simulink model "smart_home"  (R2018b)
settings: Solver=VariableStepAuto  StartTime=0.0  StopTime=intervals  RelTol=1e-3
values from neighbouring files (symbols this model uses):
  bad_q = 300    [init.m]
  good_q = 100    [init.m]
  intervals = days*stepsInDay    (= 1152)    [init.m]
  stepsInDay = 24*60/timeStep    (= 288)    [init.m]
  sunrise = floor(0.25*stepsInDay)    [init.m]
  sunset = floor(0.8*stepsInDay)    [init.m]
  T_high = 24    [init.m]
  T_low = -5    [init.m]
libraries: simulink x8
settings Model: EnablePacing=on  PacingRate=10  Creator=jf  LastModifiedBy=jf
settings SolverCC: ZeroCrossControl=DisableAll

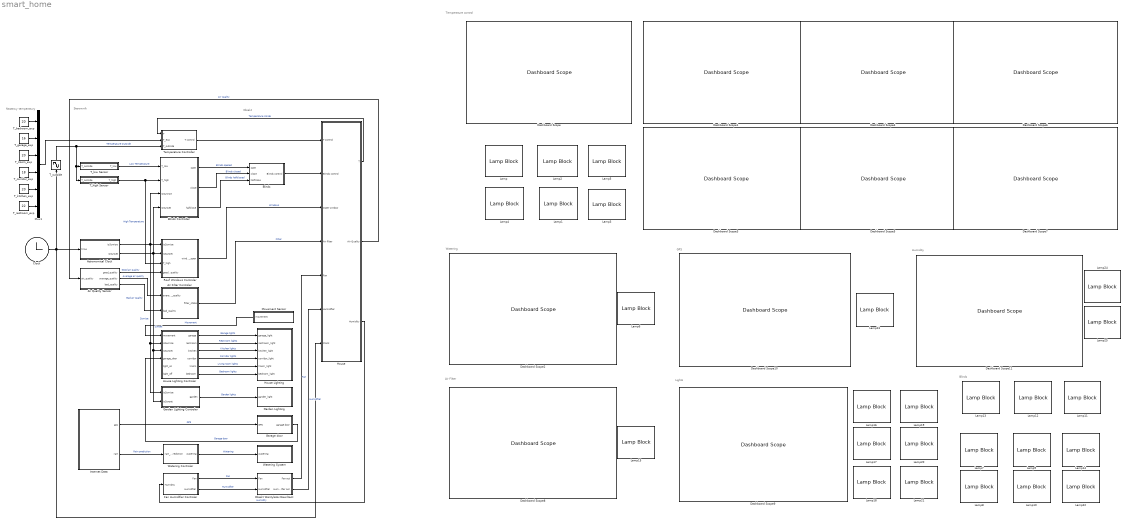
== system smart_home ==
  note: GPS
  note: Lights
  note: Air Filter
  note: Blinds
  note: Watering
  note: Temperature control
  note: Nastawy temperatury
  note: Sterownik
  note: Obiekt
  note: Humidity
  Air Filter Controler : Stateflow chart  TreatAsAtomicUnit=on
  Air Quality Sensor : Subsystem
  Astronomical Clock : Subsystem
  Blinds : Subsystem
  Blinds Controller : Stateflow chart  TreatAsAtomicUnit=on
  "Clock " : Clock
  Dashboard Scope : DashboardScope  WebBlockId=338  Ymax=30
  Dashboard Scope1 : DashboardScope  WebBlockId=352  Ymax=30
  Dashboard Scope10 : DashboardScope  WebBlockId=379  Ymin=-1  Ymax=1.5
  Dashboard Scope11 : DashboardScope  WebBlockId=384  Ymin=-1  Ymax=100
  Dashboard Scope2 : DashboardScope  WebBlockId=349  Ymin=-1  Ymax=1.5
  Dashboard Scope3 : DashboardScope  WebBlockId=353  Ymax=30
  Dashboard Scope4 : DashboardScope  WebBlockId=354  Ymax=30
  Dashboard Scope5 : DashboardScope  WebBlockId=355  Ymax=30
  Dashboard Scope6 : DashboardScope  WebBlockId=356  Ymax=30
  Dashboard Scope7 : DashboardScope  WebBlockId=357  Ymax=30
  Dashboard Scope8 : DashboardScope  WebBlockId=368  Ymin=-1  Ymax=1000
  Dashboard Scope9 : DashboardScope  WebBlockId=370  Ymin=-1  Ymax=8
  Fan Humidifier Controler : Subsystem
  Garage door : Subsystem
  Garden Lighting : Subsystem
  Garden Lighting Controler : Subsystem
  House : Subsystem
  House Lighting : Subsystem
  House Lighting Controler : Subsystem
  Internet Data : Subsystem
  Lamp : LampBlock  WebBlockId=341
  Lamp1 : LampBlock  WebBlockId=342
  Lamp10 : LampBlock  WebBlockId=361
  Lamp11 : LampBlock  WebBlockId=362
  Lamp12 : LampBlock  WebBlockId=363
  Lamp13 : LampBlock  WebBlockId=364
  Lamp14 : LampBlock  WebBlockId=366
  Lamp15 : LampBlock  WebBlockId=367
  Lamp16 : LampBlock  WebBlockId=371
  Lamp17 : LampBlock  WebBlockId=372
  Lamp18 : LampBlock  WebBlockId=373
  Lamp19 : LampBlock  WebBlockId=374
  Lamp2 : LampBlock  WebBlockId=343
  Lamp20 : LampBlock  WebBlockId=375
  Lamp21 : LampBlock  WebBlockId=376
  Lamp22 : LampBlock  WebBlockId=378
  Lamp23 : LampBlock  WebBlockId=380
  Lamp24 : LampBlock  WebBlockId=385
  Lamp25 : LampBlock  WebBlockId=387
  Lamp3 : LampBlock  WebBlockId=344
  Lamp4 : LampBlock  WebBlockId=345
  Lamp5 : LampBlock  WebBlockId=346
  Lamp6 : LampBlock  WebBlockId=350
  Lamp7 : LampBlock  WebBlockId=358
  Lamp8 : LampBlock  WebBlockId=359
  Lamp9 : LampBlock  WebBlockId=360
  Movement Sensor : Subsystem
  Mux1 : Mux  Inputs=6
  Obiekt Wentylator-Nawilzacz : Subsystem
  Roof Windows Controler : Subsystem
  T_bedroom_exp : Constant  Value=20
  T_corridor_exp : Constant  Value=18
  T_garage_exp : Constant  Value=16
  T_high Sensor : Subsystem
  T_kitchen_exp : Constant  Value=20
  T_low Sensor : Subsystem
  T_lroom_exp : Constant  Value=20
  T_outside : Sin  TimeSource=Use external signal  Amplitude=17  Bias=10  Frequency=2*pi/stepsInDay  Phase=-pi/2  SampleTime=0
  T_restroom_exp : Constant  Value=22
  Temperature Controller : Subsystem
  Watering Controler : Subsystem
  Watering System : Subsystem
  wires:
  T_high Sensor/1(T_high) -> Roof Windows Controler/3(T_high), Blinds Controller/2(T_high)  "High Temperature"
  T_garage_exp/1 -> Mux1/2
  "Clock "/1 -> Astronomical Clock/1(time), House/7(Clock), T_outside/1
  House Lighting Controler/4(corridor) -> House Lighting/4(corridor_light)  "Corridor lights"
  House Lighting Controler/5(lroom) -> House Lighting/5(lroom_light)  "Living room lights"
  Garden Lighting Controler/1(garden) -> Garden Lighting/1(garden_light)  "Garden lights"
  House Lighting Controler/1(garage) -> House Lighting/1(garage_light)  "Garage lights"
  House Lighting Controler/3(kitchen) -> House Lighting/3(kitchen_light)  "Kitchen lights"
  T_corridor_exp/1 -> Mux1/4
  T_restroom_exp/1 -> Mux1/6
  T_lroom_exp/1 -> Mux1/3
  T_bedroom_exp/1 -> Mux1/1
  T_kitchen_exp/1 -> Mux1/5
  House Lighting Controler/6(bedroom) -> House Lighting/6(bedroom_light)  "Bedroom lights"
  House Lighting Controler/2(restroom) -> House Lighting/2(restroom_light)  "Restroom lights"
  T_low Sensor/1(T_low) -> Blinds Controller/1(T_low)  "Low Temperature"
  Air Quality Sensor/1(good_quality) -> Roof Windows Controler/4(good_air_quality)  "Good air quality"
  Watering Controler/1(watering) -> Watering System/1(watering)  "Watering"
  Air Quality Sensor/2(avarage_quality) -> Air Filter Controler/1(average_quality)  "Avarage air quality"
  Air Quality Sensor/3(bad_quality) -> Air Filter Controler/2(bad_quality)  "Bad air quality"
  Blinds Controller/1(open) -> Blinds/1(open)  "Blinds opened"
  Blinds Controller/2(close) -> Blinds/2(close)  "Blinds closed"
  Blinds Controller/3(halfclose) -> Blinds/3(halfclose)  "Blinds halfclosed"
  Blinds/1(Blinds control) -> House/2(Blinds control)
  Roof Windows Controler/1(window_open) -> House/3(Open window)  "Windows"
  Air Filter Controler/1(filter_state) -> House/4(Air filter)  "Filter"
  House/1(T) -> Temperature Controller/1(T)  "Temperature inside"
  Temperature Controller/1(T control) -> House/1(T control)
  Mux1/1 -> Temperature Controller/2(T_exp)
  T_outside/1 -> T_high Sensor/1(T_outside), T_low Sensor/1(T_outside), Temperature Controller/3(T_outside)  "Temperature Outside"
  Internet Data/2(rain) -> Watering Controler/1(rain_prediction)  "Rain prediction"
  Internet Data/1(gps) -> Garage door/1(GPS)  "GPS"
  Astronomical Clock/1(isSunrise) -> Roof Windows Controler/1(isSunrise), Garden Lighting Controler/1(isSunrise), House Lighting Controler/2(isSunrise), Blinds Controller/3(isSunrise)  "Sunrise"
  Astronomical Clock/2(isSunset) -> House Lighting Controler/3(isSunset), Garden Lighting Controler/2(isSunset), Blinds Controller/4(isSunset), Roof Windows Controler/2(isSunset)  "Sunset"
  Movement Sensor/1(movement) -> House Lighting Controler/1(movement)  "Movement"
  House/2(Air Quality) -> Air Quality Sensor/1(air_quality)  "Air quality"
  Garage door/1(garage door) -> House Lighting Controler/4(garage_door)  "Garage door"
  Fan Humidifier Controler/1(Fan) -> Obiekt Wentylator-Nawilzacz/1(Fan)  "Fan"
  Fan Humidifier Controler/2(Humidifier) -> Obiekt Wentylator-Nawilzacz/2(Humidifier)  "Humidifier"
  House/3(Humidity) -> Fan Humidifier Controler/1(Humidity)  "Humidity"
  Obiekt Wentylator-Nawilzacz/1(Fan out) -> House/5(Fan)  "Fan"
  Obiekt Wentylator-Nawilzacz/2(Humidifier out) -> House/6(Humidifier)  "Humidifier"

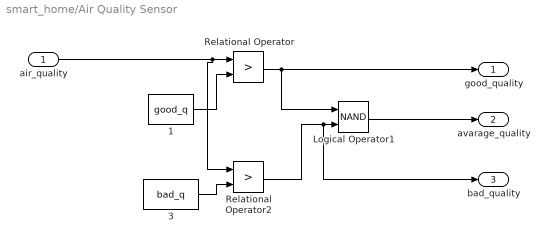
== system smart_home/Air Quality Sensor ==
  air_quality : Inport
  1 : Constant  Value=good_q
  3 : Constant  Value=bad_q
  Logical Operator1 : Logic  Operator=NAND  AllPortsSameDT=off  OutDataTypeStr=boolean
  Relational Operator : RelationalOperator  Operator=>  OutDataTypeStr=boolean  RndMeth=Simplest
  Relational Operator2 : RelationalOperator  Operator=>  OutDataTypeStr=boolean  RndMeth=Simplest
  good_quality : Outport
  avarage_quality : Outport  Port=2
  bad_quality : Outport  Port=3
  wires:
  3/1 -> Relational Operator2/2
  Relational Operator/1 -> Logical Operator1/1, good_quality/1
  1/1 -> Relational Operator/2
  Relational Operator2/1 -> Logical Operator1/2, bad_quality/1
  Logical Operator1/1 -> avarage_quality/1
  air_quality/1 -> Relational Operator/1, Relational Operator2/1

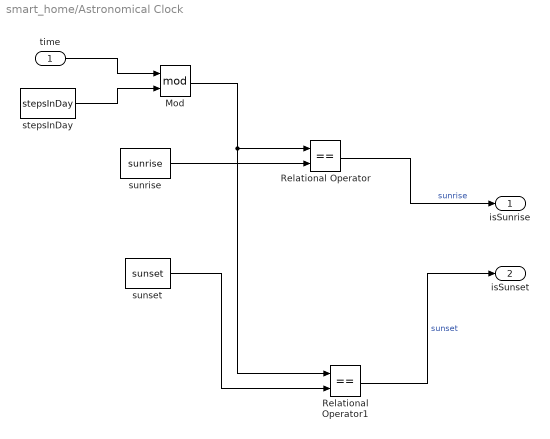
== system smart_home/Astronomical Clock ==
  time : Inport
  Mod : Math  Operator=mod  SaturateOnIntegerOverflow=on
  Relational Operator : RelationalOperator  Operator===  OutDataTypeStr=boolean  RndMeth=Simplest
  Relational Operator1 : RelationalOperator  Operator===  OutDataTypeStr=boolean  RndMeth=Simplest
  stepsInDay : Constant  Value=stepsInDay
  sunrise : Constant  Value=sunrise
  sunset : Constant  Value=sunset
  isSunrise : Outport
  isSunset : Outport  Port=2
  wires:
  Relational Operator1/1 -> isSunset/1  "sunset"
  sunrise/1 -> Relational Operator/2
  Relational Operator/1 -> isSunrise/1  "sunrise"
  sunset/1 -> Relational Operator1/2
  time/1 -> Mod/1
  Mod/1 -> Relational Operator1/1, Relational Operator/1
  stepsInDay/1 -> Mod/2

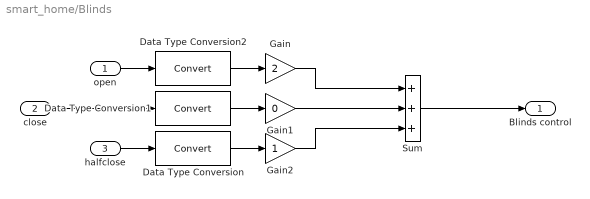
== system smart_home/Blinds ==
  open : Inport
  close : Inport  Port=2
  halfclose : Inport  Port=3
  Data Type Conversion : DataTypeConversion
  Data Type Conversion1 : DataTypeConversion
  Data Type Conversion2 : DataTypeConversion
  Gain : Gain  Gain=2
  Gain1 : Gain  Gain=0
  Gain2 : Gain
  Sum : Sum  Inputs=+++
  Blinds control : Outport
  wires:
  Gain/1 -> Sum/1
  halfclose/1 -> Data Type Conversion/1
  Gain1/1 -> Sum/2
  close/1 -> Data Type Conversion1/1
  Gain2/1 -> Sum/3
  open/1 -> Data Type Conversion2/1
  Sum/1 -> Blinds control/1
  Data Type Conversion/1 -> Gain2/1
  Data Type Conversion1/1 -> Gain1/1
  Data Type Conversion2/1 -> Gain/1

== system smart_home/Fan Humidifier Controler ==
  Humidity : Inport
  Sterowanie nawilzaczem : Relay  OnSwitchValue=60  OffSwitchValue=50  OnOutputValue=0  OffOutputValue=1
  Sterowanie wentylatorem : Relay  OnSwitchValue=70  OffSwitchValue=60
  Fan : Outport
  Humidifier : Outport  Port=2
  wires:
  Sterowanie nawilzaczem/1 -> Humidifier/1
  Humidity/1 -> Sterowanie wentylatorem/1, Sterowanie nawilzaczem/1
  Sterowanie wentylatorem/1 -> Fan/1

== system smart_home/Garage door ==
  GPS : Inport
  Chart : Stateflow chart  TreatAsAtomicUnit=on
  Constant : Constant  Value=5
  Data Type Conversion : DataTypeConversion
  Ground : Ground
  if : simulink/Logic and Bit Operations/Compare To Constant  relop=>=  const=0.5  OutDataTypeStr=boolean
  garage door : Outport
  wires:
  GPS/1 -> if/1
  Chart/1(x) -> garage door/1
  Constant/1 -> Chart/3(ts)
  Data Type Conversion/1 -> Chart/2(u)
  if/1 -> Data Type Conversion/1
  Ground/1 -> Chart/1(y)

== system smart_home/Garden Lighting ==
  garden_light : Inport
  To Workspace : ToWorkspace  VariableName=garden_light  SaveFormat=Timeseries  SampleTime=-1
  wires:
  garden_light/1 -> To Workspace/1

== system smart_home/Garden Lighting Controler ==
  isSunrise : Inport
  isSunset : Inport  Port=2
  Chart6 : Stateflow chart  TreatAsAtomicUnit=on
  garden : Outport
  wires:
  isSunrise/1 -> Chart6/1(isSunrise)
  Chart6/1(sunState) -> garden/1
  isSunset/1 -> Chart6/2(isSunset)

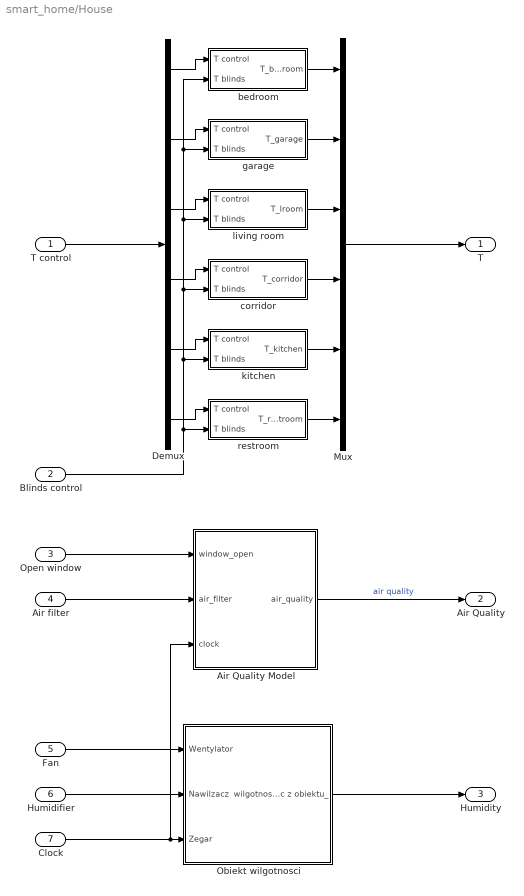
== system smart_home/House ==
  T control : Inport
  Blinds control : Inport  Port=2
  Open window : Inport  Port=3
  Air filter : Inport  Port=4
  Fan : Inport  Port=5
  Humidifier : Inport  Port=6
  Clock : Inport  Port=7
  Air Quality Model : Subsystem
  Demux : Demux  Outputs=6
  Mux : Mux  Inputs=6
  Obiekt wilgotnosci : Subsystem
  bedroom : Subsystem
  corridor : Subsystem
  garage : Subsystem
  kitchen : Subsystem
  living room : Subsystem
  restroom : Subsystem
  T : Outport
  Air Quality : Outport  Port=2
  Humidity : Outport  Port=3
  wires:
  T control/1 -> Demux/1
  Blinds control/1 -> restroom/2(T blinds), kitchen/2(T blinds), corridor/2(T blinds), living room/2(T blinds), garage/2(T blinds), bedroom/2(T blinds)
  Demux/6 -> restroom/1(T control)
  Demux/3 -> living room/1(T control)
  bedroom/1(T_bedroom) -> Mux/1
  Demux/2 -> garage/1(T control)
  living room/1(T_lroom) -> Mux/3
  garage/1(T_garage) -> Mux/2
  restroom/1(T_restroom) -> Mux/6
  kitchen/1(T_kitchen) -> Mux/5
  Demux/1 -> bedroom/1(T control)
  Demux/4 -> corridor/1(T control)
  corridor/1(T_corridor) -> Mux/4
  Demux/5 -> kitchen/1(T control)
  Mux/1 -> T/1
  Air Quality Model/1(air_quality) -> Air Quality/1  "air quality"
  Open window/1 -> Air Quality Model/1(window_open)
  Air filter/1 -> Air Quality Model/2(air_filter)
  Obiekt wilgotnosci/1(wilgotnosc z obiektu_) -> Humidity/1
  Clock/1 -> Air Quality Model/3(clock), Obiekt wilgotnosci/3(Zegar)
  Humidifier/1 -> Obiekt wilgotnosci/2(Nawilzacz)
  Fan/1 -> Obiekt wilgotnosci/1(Wentylator)

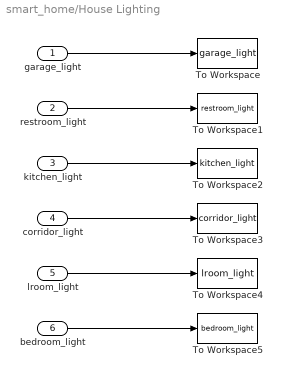
== system smart_home/House Lighting ==
  garage_light : Inport
  restroom_light : Inport  Port=2
  kitchen_light : Inport  Port=3
  corridor_light : Inport  Port=4
  lroom_light : Inport  Port=5
  bedroom_light : Inport  Port=6
  To Workspace : ToWorkspace  VariableName=garage_light  SaveFormat=Timeseries  SampleTime=-1
  To Workspace1 : ToWorkspace  VariableName=restroom_light  SaveFormat=Timeseries  SampleTime=-1
  To Workspace2 : ToWorkspace  VariableName=kitchen_light  SaveFormat=Timeseries  SampleTime=-1
  To Workspace3 : ToWorkspace  VariableName=corridor_light  SaveFormat=Timeseries  SampleTime=-1
  To Workspace4 : ToWorkspace  VariableName=lroom_light  SaveFormat=Timeseries  SampleTime=-1
  To Workspace5 : ToWorkspace  VariableName=bedroom_light  SaveFormat=Timeseries  SampleTime=-1
  wires:
  bedroom_light/1 -> To Workspace5/1
  garage_light/1 -> To Workspace/1
  corridor_light/1 -> To Workspace3/1
  restroom_light/1 -> To Workspace1/1
  lroom_light/1 -> To Workspace4/1
  kitchen_light/1 -> To Workspace2/1

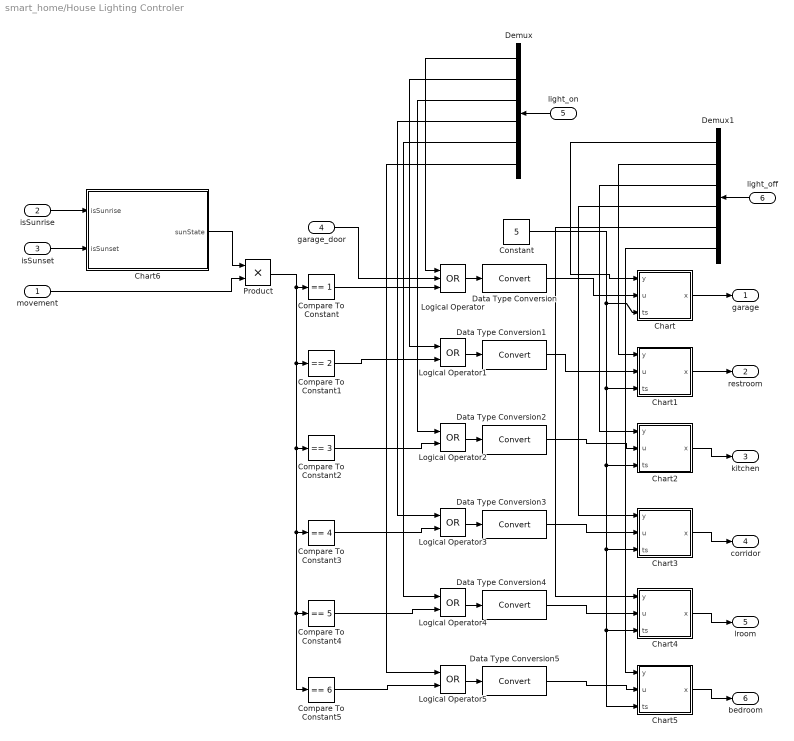
== system smart_home/House Lighting Controler ==
  movement : Inport
  isSunrise : Inport  Port=2
  isSunset : Inport  Port=3
  garage_door : Inport  Port=4
  light_on : Inport  Port=5
  light_off : Inport  Port=6
  Chart : Stateflow chart  TreatAsAtomicUnit=on
  Chart1 : Stateflow chart  TreatAsAtomicUnit=on
  Chart2 : Stateflow chart  TreatAsAtomicUnit=on
  Chart3 : Stateflow chart  TreatAsAtomicUnit=on
  Chart4 : Stateflow chart  TreatAsAtomicUnit=on
  Chart5 : Stateflow chart  TreatAsAtomicUnit=on
  Chart6 : Stateflow chart  TreatAsAtomicUnit=on
  Compare To Constant : simulink/Logic and Bit Operations/Compare To Constant  relop===  const=1  OutDataTypeStr=boolean
  Compare To Constant1 : simulink/Logic and Bit Operations/Compare To Constant  relop===  const=2  OutDataTypeStr=boolean
  Compare To Constant2 : simulink/Logic and Bit Operations/Compare To Constant  relop===  const=3  OutDataTypeStr=boolean
  Compare To Constant3 : simulink/Logic and Bit Operations/Compare To Constant  relop===  const=4  OutDataTypeStr=boolean
  Compare To Constant4 : simulink/Logic and Bit Operations/Compare To Constant  relop===  const=5  OutDataTypeStr=boolean
  Compare To Constant5 : simulink/Logic and Bit Operations/Compare To Constant  relop===  const=6  OutDataTypeStr=boolean
  Constant : Constant  Value=5
  Data Type Conversion{,1..5} (6 alike) : DataTypeConversion
  Demux : Demux  Outputs=6
  Demux1 : Demux  Outputs=6
  Logical Operator : Logic  Operator=OR  Inputs=3  AllPortsSameDT=off  OutDataTypeStr=boolean
  Logical Operator{1..5} (5 alike) : Logic  Operator=OR  AllPortsSameDT=off  OutDataTypeStr=boolean
  Product : Product
  garage : Outport
  restroom : Outport  Port=2
  kitchen : Outport  Port=3
  corridor : Outport  Port=4
  lroom : Outport  Port=5
  bedroom : Outport  Port=6
  wires:
  light_off/1 -> Demux1/1
  Demux1/6 -> Chart5/1(y)
  Demux1/5 -> Chart4/1(y)
  Demux1/4 -> Chart3/1(y)
  Demux1/3 -> Chart2/1(y)
  Demux1/2 -> Chart1/1(y)
  Demux1/1 -> Chart/1(y)
  light_on/1 -> Demux/1
  Compare To Constant5/1 -> Logical Operator5/2
  Compare To Constant4/1 -> Logical Operator4/2
  Compare To Constant3/1 -> Logical Operator3/2
  Compare To Constant2/1 -> Logical Operator2/2
  Demux/6 -> Logical Operator5/1
  Demux/5 -> Logical Operator4/1
  Demux/4 -> Logical Operator3/1
  Demux/3 -> Logical Operator2/1
  Logical Operator5/1 -> Data Type Conversion5/1
  Logical Operator4/1 -> Data Type Conversion4/1
  Logical Operator3/1 -> Data Type Conversion3/1
  Logical Operator2/1 -> Data Type Conversion2/1
  Demux/2 -> Logical Operator1/1
  Compare To Constant1/1 -> Logical Operator1/2
  Logical Operator1/1 -> Data Type Conversion1/1
  Demux/1 -> Logical Operator/1
  Chart5/1(x) -> bedroom/1
  Chart4/1(x) -> lroom/1
  Chart3/1(x) -> corridor/1
  Chart2/1(x) -> kitchen/1
  Chart1/1(x) -> restroom/1
  Chart/1(x) -> garage/1
  garage_door/1 -> Logical Operator/2
  Logical Operator/1 -> Data Type Conversion/1
  Compare To Constant/1 -> Logical Operator/3
  Product/1 -> Compare To Constant/1, Compare To Constant1/1, Compare To Constant2/1, Compare To Constant3/1, Compare To Constant4/1, Compare To Constant5/1
  Chart6/1(sunState) -> Product/1
  isSunrise/1 -> Chart6/1(isSunrise)
  isSunset/1 -> Chart6/2(isSunset)
  Data Type Conversion5/1 -> Chart5/2(u)
  Data Type Conversion4/1 -> Chart4/2(u)
  Data Type Conversion3/1 -> Chart3/2(u)
  Data Type Conversion2/1 -> Chart2/2(u)
  Data Type Conversion1/1 -> Chart1/2(u)
  Data Type Conversion/1 -> Chart/2(u)
  Constant/1 -> Chart4/3(ts), Chart5/3(ts), Chart3/3(ts), Chart2/3(ts), Chart1/3(ts), Chart/3(ts)
  movement/1 -> Product/2

== system smart_home/Internet Data ==
  From Workspace1 : FromWorkspace  VariableName=inhabitant_gps  SampleTime=0
  From Workspace2 : FromWorkspace  VariableName=rain_prediction  SampleTime=0
  gps : Outport
  rain : Outport  Port=2
  wires:
  From Workspace1/1 -> gps/1
  From Workspace2/1 -> rain/1

== system smart_home/Movement Sensor ==
  From Workspace : FromWorkspace  VariableName=inhabitant_movement  SampleTime=0
  movement : Outport
  wires:
  From Workspace/1 -> movement/1

== system smart_home/Obiekt Wentylator-Nawilzacz ==
  Fan : Inport
  Humidifier : Inport  Port=2
  Nastawa Nawilzacza : Gain  Gain=30
  Nastawa Wentylatora : Gain  Gain=-30
  Fan out : Outport
  Humidifier out : Outport  Port=2
  wires:
  Nastawa Wentylatora/1 -> Fan out/1
  Nastawa Nawilzacza/1 -> Humidifier out/1
  Fan/1 -> Nastawa Wentylatora/1
  Humidifier/1 -> Nastawa Nawilzacza/1

== system smart_home/Roof Windows Controler ==
  isSunrise : Inport
  isSunset : Inport  Port=2
  T_high : Inport  Port=3
  good_air_quality : Inport  Port=4
  Chart6 : Stateflow chart  TreatAsAtomicUnit=on
  Logical Operator : Logic  Inputs=3  AllPortsSameDT=off  OutDataTypeStr=boolean
  window_open : Outport
  wires:
  good_air_quality/1 -> Logical Operator/3
  T_high/1 -> Logical Operator/2
  Chart6/1(sunState) -> Logical Operator/1
  Logical Operator/1 -> window_open/1
  isSunset/1 -> Chart6/2(isSunset)
  isSunrise/1 -> Chart6/1(isSunrise)

== system smart_home/T_high Sensor ==
  T_outside : Inport
  Relational Operator : RelationalOperator  Operator=>  OutDataTypeStr=boolean  RndMeth=Simplest
  T_cap_H : Constant  Value=T_high
  T_high : Outport
  wires:
  T_outside/1 -> Relational Operator/1
  T_cap_H/1 -> Relational Operator/2
  Relational Operator/1 -> T_high/1  "T_cap_H"

== system smart_home/T_low Sensor ==
  T_outside : Inport
  Relational Operator1 : RelationalOperator  Operator=<  OutDataTypeStr=boolean  RndMeth=Simplest
  T_cap_L : Constant  Value=T_low
  T_low : Outport
  wires:
  T_cap_L/1 -> Relational Operator1/2
  Relational Operator1/1 -> T_low/1  "T_cap_L"
  T_outside/1 -> Relational Operator1/1

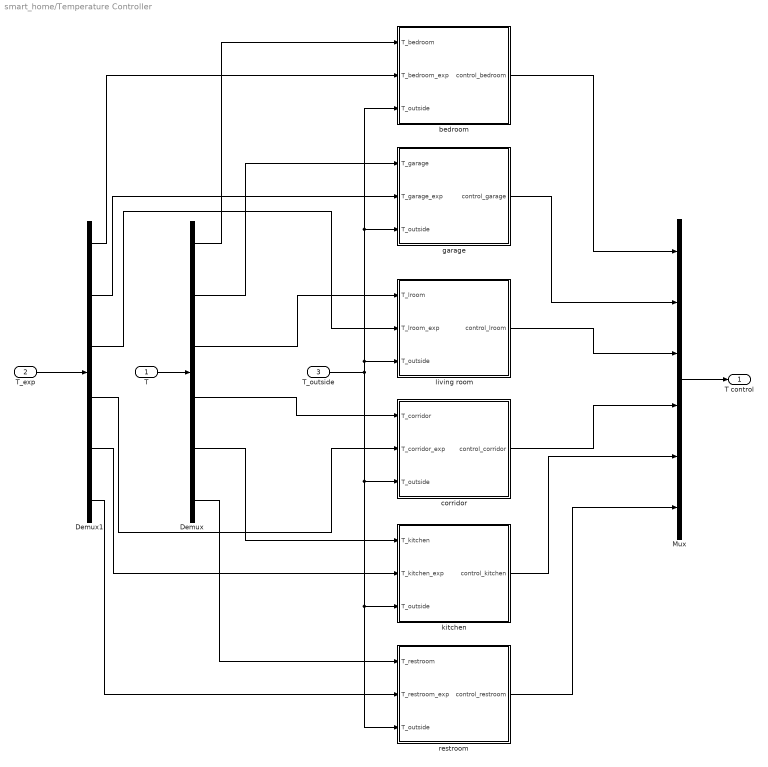
== system smart_home/Temperature Controller ==
  T : Inport
  T_exp : Inport  Port=2
  T_outside : Inport  Port=3
  Demux : Demux  Outputs=6
  Demux1 : Demux  Outputs=6
  Mux : Mux  Inputs=6
  bedroom : Subsystem
  corridor : Subsystem
  garage : Subsystem
  kitchen : Subsystem
  living room : Subsystem
  restroom : Subsystem
  T control : Outport
  wires:
  T/1 -> Demux/1
  T_exp/1 -> Demux1/1
  Demux/1 -> bedroom/1(T_bedroom)
  Demux/2 -> garage/1(T_garage)
  Demux/3 -> living room/1(T_lroom)
  Demux/4 -> corridor/1(T_corridor)
  Demux/5 -> kitchen/1(T_kitchen)
  Demux/6 -> restroom/1(T_restroom)
  Demux1/1 -> bedroom/2(T_bedroom_exp)
  Demux1/2 -> garage/2(T_garage_exp)
  Demux1/3 -> living room/2(T_lroom_exp)
  Demux1/4 -> corridor/2(T_corridor_exp)
  Demux1/5 -> kitchen/2(T_kitchen_exp)
  Demux1/6 -> restroom/2(T_restroom_exp)
  bedroom/1(control_bedroom) -> Mux/1
  garage/1(control_garage) -> Mux/2
  living room/1(control_lroom) -> Mux/3
  corridor/1(control_corridor) -> Mux/4
  kitchen/1(control_kitchen) -> Mux/5
  restroom/1(control_restroom) -> Mux/6
  Mux/1 -> T control/1
  T_outside/1 -> living room/3(T_outside), bedroom/3(T_outside), garage/3(T_outside), restroom/3(T_outside), kitchen/3(T_outside), corridor/3(T_outside)

== system smart_home/Watering Controler ==
  rain_prediction : Inport
  Chart : Stateflow chart  TreatAsAtomicUnit=on
  Compare To Constant : simulink/Logic and Bit Operations/Compare To Constant  relop===  const=0  OutDataTypeStr=boolean
  Constant : Constant  Value=4320
  Data Type Conversion : DataTypeConversion
  Ground : Ground
  watering : Outport
  wires:
  Chart/1(x) -> watering/1
  Constant/1 -> Chart/3(ts)
  rain_prediction/1 -> Compare To Constant/1
  Compare To Constant/1 -> Data Type Conversion/1
  Data Type Conversion/1 -> Chart/2(u)
  Ground/1 -> Chart/1(y)

== system smart_home/Watering System ==
  watering : Inport
  To Workspace : ToWorkspace  VariableName=watering_state  SaveFormat=Timeseries  SampleTime=-1
  wires:
  watering/1 -> To Workspace/1

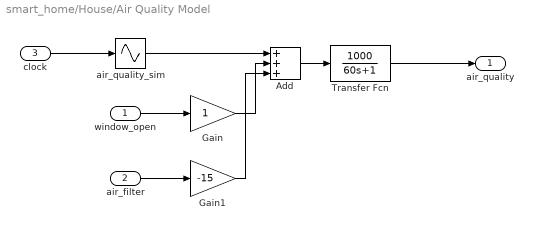
== system smart_home/House/Air Quality Model ==
  window_open : Inport
  air_filter : Inport  Port=2
  clock : Inport  Port=3
  Add : Sum  Inputs=+++
  Gain : Gain
  Gain1 : Gain  Gain=-15
  Transfer Fcn : TransferFcn  Numerator=[1000]  Denominator=[60 1]
  air_quality_sim : Sin  TimeSource=Use external signal  Amplitude=0.4  Bias=0.6  Frequency=2*pi/stepsInDay  Phase=-pi/2  SampleTime=0
  air_quality : Outport
  wires:
  Transfer Fcn/1 -> air_quality/1
  Gain/1 -> Add/2
  air_filter/1 -> Gain1/1
  Add/1 -> Transfer Fcn/1
  Gain1/1 -> Add/3
  air_quality_sim/1 -> Add/1
  window_open/1 -> Gain/1
  clock/1 -> air_quality_sim/1

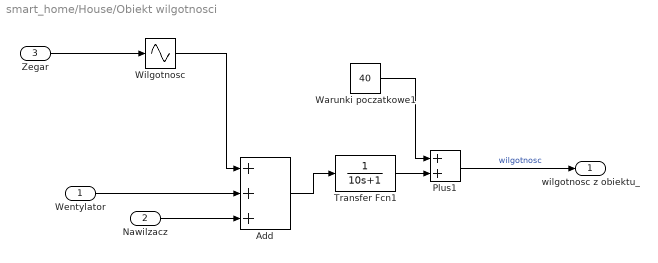
== system smart_home/House/Obiekt wilgotnosci ==
  Wentylator : Inport
  Nawilzacz : Inport  Port=2
  Zegar : Inport  Port=3
  Add : Sum  Inputs=+++
  Plus1 : Sum
  Transfer Fcn1 : TransferFcn  Denominator=[10 1]
  Warunki poczatkowe1 : Constant  Value=40
  Wilgotnosc : Sin  TimeSource=Use external signal  Amplitude=20  Bias=20  Frequency=2*pi/intervals  Phase=-pi/2  SampleTime=0
  wilgotnosc z obiektu_ : Outport
  wires:
  Warunki poczatkowe1/1 -> Plus1/1
  Wentylator/1 -> Add/2
  Zegar/1 -> Wilgotnosc/1
  Transfer Fcn1/1 -> Plus1/2
  Add/1 -> Transfer Fcn1/1
  Nawilzacz/1 -> Add/3
  Plus1/1 -> wilgotnosc z obiektu_/1  "wilgotnosc"
  Wilgotnosc/1 -> Add/1

== system smart_home/House/bedroom ==
  T control : Inport
  T blinds : Inport  Port=2
  Sum : Sum  Inputs=|++
  temperature model : TransferFcn  Denominator=[30 1]
  temperature model1 : TransferFcn  Denominator=[15 1]
  T_bedroom : Outport
  wires:
  T control/1 -> temperature model/1
  T blinds/1 -> temperature model1/1
  temperature model/1 -> Sum/1
  Sum/1 -> T_bedroom/1
  temperature model1/1 -> Sum/2

== system smart_home/House/corridor ==
  T control : Inport
  T blinds : Inport  Port=2
  Sum : Sum  Inputs=|++
  corridor temperature model : TransferFcn  Denominator=[32 1]
  corridor temperature model1 : TransferFcn  Denominator=[15 1]
  T_corridor : Outport
  wires:
  corridor temperature model/1 -> Sum/1
  T control/1 -> corridor temperature model/1
  T blinds/1 -> corridor temperature model1/1
  Sum/1 -> T_corridor/1
  corridor temperature model1/1 -> Sum/2

== system smart_home/House/garage ==
  T control : Inport
  T blinds : Inport  Port=2
  Sum : Sum  Inputs=|++
  temperature model : TransferFcn  Denominator=[18 1]
  temperature model1 : TransferFcn  Denominator=[15 1]
  T_garage : Outport
  wires:
  T control/1 -> temperature model/1
  temperature model/1 -> Sum/1
  temperature model1/1 -> Sum/2
  T blinds/1 -> temperature model1/1
  Sum/1 -> T_garage/1

== system smart_home/House/kitchen ==
  T control : Inport
  T blinds : Inport  Port=2
  Sum : Sum  Inputs=|++
  kitchen temperature model : TransferFcn  Denominator=[32 1]
  kitchen temperature model1 : TransferFcn  Denominator=[15 1]
  T_kitchen : Outport
  wires:
  kitchen temperature model/1 -> Sum/1
  T control/1 -> kitchen temperature model/1
  T blinds/1 -> kitchen temperature model1/1
  Sum/1 -> T_kitchen/1
  kitchen temperature model1/1 -> Sum/2

== system smart_home/House/living room ==
  T control : Inport
  T blinds : Inport  Port=2
  Sum : Sum  Inputs=|++
  living room blinds temperature model : TransferFcn  Denominator=[15 1]
  living room temperature model : TransferFcn  Denominator=[25 1]
  T_lroom : Outport
  wires:
  T control/1 -> living room temperature model/1
  T blinds/1 -> living room blinds temperature model/1
  living room temperature model/1 -> Sum/1
  Sum/1 -> T_lroom/1
  living room blinds temperature model/1 -> Sum/2

== system smart_home/House/restroom ==
  T control : Inport
  T blinds : Inport  Port=2
  Sum : Sum  Inputs=|++
  kitchen temperature model1 : TransferFcn  Denominator=[15 1]
  restroom temperature model : TransferFcn  Denominator=[32 1]
  T_restroom : Outport
  wires:
  restroom temperature model/1 -> Sum/1
  T control/1 -> restroom temperature model/1
  T blinds/1 -> kitchen temperature model1/1
  Sum/1 -> T_restroom/1
  kitchen temperature model1/1 -> Sum/2

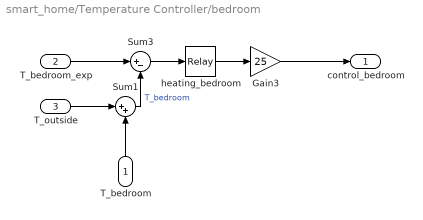
== system smart_home/Temperature Controller/bedroom ==
  T_bedroom : Inport
  T_bedroom_exp : Inport  Port=2
  T_outside : Inport  Port=3
  Gain3 : Gain  Gain=25
  Sum1 : Sum  Inputs=|++
  Sum3 : Sum  Inputs=|+-
  heating_bedroom : Relay  OnSwitchValue=2  OffSwitchValue=-2
  control_bedroom : Outport
  wires:
  T_bedroom_exp/1 -> Sum3/1
  Sum1/1 -> Sum3/2  "T_bedroom"
  Gain3/1 -> control_bedroom/1
  T_bedroom/1 -> Sum1/2
  Sum3/1 -> heating_bedroom/1
  heating_bedroom/1 -> Gain3/1
  T_outside/1 -> Sum1/1

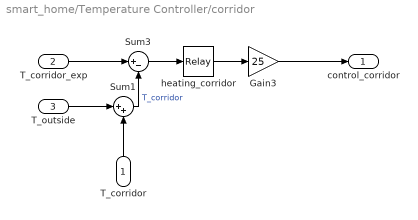
== system smart_home/Temperature Controller/corridor ==
  T_corridor : Inport
  T_corridor_exp : Inport  Port=2
  T_outside : Inport  Port=3
  Gain3 : Gain  Gain=25
  Sum1 : Sum  Inputs=|++
  Sum3 : Sum  Inputs=|+-
  heating_corridor : Relay  OnSwitchValue=2  OffSwitchValue=-2
  control_corridor : Outport
  wires:
  T_corridor_exp/1 -> Sum3/1
  Sum1/1 -> Sum3/2  "T_corridor"
  Gain3/1 -> control_corridor/1
  T_corridor/1 -> Sum1/2
  Sum3/1 -> heating_corridor/1
  heating_corridor/1 -> Gain3/1
  T_outside/1 -> Sum1/1

== system smart_home/Temperature Controller/garage ==
  T_garage : Inport
  T_garage_exp : Inport  Port=2
  T_outside : Inport  Port=3
  Gain3 : Gain  Gain=25
  Sum1 : Sum  Inputs=|++
  Sum3 : Sum  Inputs=|+-
  heating_garage : Relay  OnSwitchValue=2  OffSwitchValue=-2
  control_garage : Outport
  wires:
  T_garage_exp/1 -> Sum3/1
  Sum1/1 -> Sum3/2  "T_garage"
  Gain3/1 -> control_garage/1
  T_garage/1 -> Sum1/2
  Sum3/1 -> heating_garage/1
  heating_garage/1 -> Gain3/1
  T_outside/1 -> Sum1/1

== system smart_home/Temperature Controller/kitchen ==
  T_kitchen : Inport
  T_kitchen_exp : Inport  Port=2
  T_outside : Inport  Port=3
  Gain3 : Gain  Gain=25
  Sum1 : Sum  Inputs=|++
  Sum3 : Sum  Inputs=|+-
  heating_kitchen : Relay  OnSwitchValue=2  OffSwitchValue=-2
  control_kitchen : Outport
  wires:
  T_kitchen_exp/1 -> Sum3/1
  Sum1/1 -> Sum3/2  "T_kitchen"
  Gain3/1 -> control_kitchen/1
  T_kitchen/1 -> Sum1/2
  Sum3/1 -> heating_kitchen/1
  heating_kitchen/1 -> Gain3/1
  T_outside/1 -> Sum1/1

== system smart_home/Temperature Controller/living room ==
  T_lroom : Inport
  T_lroom_exp : Inport  Port=2
  T_outside : Inport  Port=3
  Gain3 : Gain  Gain=25
  Sum1 : Sum  Inputs=|++
  Sum3 : Sum  Inputs=|+-
  heating_lroom : Relay  OnSwitchValue=2  OffSwitchValue=-2
  control_lroom : Outport
  wires:
  T_lroom_exp/1 -> Sum3/1
  Sum1/1 -> Sum3/2  "T_lroom"
  Gain3/1 -> control_lroom/1
  T_lroom/1 -> Sum1/2
  Sum3/1 -> heating_lroom/1
  heating_lroom/1 -> Gain3/1
  T_outside/1 -> Sum1/1

== system smart_home/Temperature Controller/restroom ==
  T_restroom : Inport
  T_restroom_exp : Inport  Port=2
  T_outside : Inport  Port=3
  Gain3 : Gain  Gain=25
  Sum1 : Sum  Inputs=|++
  Sum3 : Sum  Inputs=|+-
  heating_restroom : Relay  OnSwitchValue=2  OffSwitchValue=-2
  control_restroom : Outport
  wires:
  T_restroom_exp/1 -> Sum3/1
  Sum1/1 -> Sum3/2  "T_restroom"
  Gain3/1 -> control_restroom/1
  T_restroom/1 -> Sum1/2
  Sum3/1 -> heating_restroom/1
  heating_restroom/1 -> Gain3/1
  T_outside/1 -> Sum1/1

== stateflow chart smart_home/House Lighting Controler/Chart ==
  settings: updateMethod=DISCRETE  sampleTime=1  executeAtInitialization=1
  state Idle
    x=0;
    t1=ts/timeStep;
  state State1
    x=1;
  state Wait
  (default) -> Idle
  Idle -> Idle [order 2]
  Wait -> Idle [order 2] : after(t1,'sec')
  Idle -> State1 [order 1] : [u>=1]
  State1 -> Idle [order 2] : [y==1]
  State1 -> Wait [order 1] : [u==0]
  Wait -> State1 [order 1] : [u==1]
  data: y input; u input; x output; ts input; timeStep constant double; t1 local

== stateflow chart smart_home/House Lighting Controler/Chart1 ==
  settings: updateMethod=DISCRETE  sampleTime=1  executeAtInitialization=1
  state Idle
    x=0;
    t1=ts/timeStep;
  state State1
    x=1;
  state Wait
  (default) -> Idle
  Idle -> Idle [order 2]
  Wait -> Idle [order 2] : after(t1,'sec')
  Idle -> State1 [order 1] : [u>=1]
  State1 -> Idle [order 2] : [y==1]
  State1 -> Wait [order 1] : [u==0]
  Wait -> State1 [order 1] : [u==1]
  data: y input; u input; x output; ts input; timeStep constant double; t1 local

== stateflow chart smart_home/Blinds Controller ==
  settings: executeAtInitialization=1
  state State
    state Night
      state Open
        open = true;
        halfclose = false;
        close = false;
      state Close
        close = true;
        open = false;
        halfclose = false;
      (default) -> Close
      Close -> State.Night.Open : [T_low]
      State.Night.Open -> Close : [~T_low]
    state Day
      state HalfClose
        halfclose = true;
        open = false;
        close = false;
      state Open
        open = true;
        halfclose = false;
        close = false;
      (default) -> State.Day.Open
      State.Day.Open -> HalfClose : [T_high]
      HalfClose -> State.Day.Open : [~T_high]
    (default) -> Night
    Day -> Night : [isSunset]
    Night -> Day : [isSunrise]
  data: T_low input; T_high input; isSunrise input; isSunset input; open output boolean; close output boolean; halfclose output boolean

== stateflow chart smart_home/House Lighting Controler/Chart2 ==
  settings: updateMethod=DISCRETE  sampleTime=1  executeAtInitialization=1
  state Idle
    x=0;
    t1=ts/timeStep;
  state State1
    x=1;
  state Wait
  (default) -> Idle
  Idle -> Idle [order 2]
  Wait -> Idle [order 2] : after(t1,'sec')
  Idle -> State1 [order 1] : [u>=1]
  State1 -> Idle [order 2] : [y==1]
  State1 -> Wait [order 1] : [u==0]
  Wait -> State1 [order 1] : [u==1]
  data: y input; u input; x output; ts input; timeStep constant double; t1 local

== stateflow chart smart_home/House Lighting Controler/Chart3 ==
  settings: updateMethod=DISCRETE  sampleTime=1  executeAtInitialization=1
  state Idle
    x=0;
    t1=ts/timeStep;
  state State1
    x=1;
  state Wait
  (default) -> Idle
  Idle -> Idle [order 2]
  Wait -> Idle [order 2] : after(t1,'sec')
  Idle -> State1 [order 1] : [u>=1]
  State1 -> Idle [order 2] : [y==1]
  State1 -> Wait [order 1] : [u==0]
  Wait -> State1 [order 1] : [u==1]
  data: y input; u input; x output; ts input; timeStep constant double; t1 local

== stateflow chart smart_home/House Lighting Controler/Chart4 ==
  settings: updateMethod=DISCRETE  sampleTime=1  executeAtInitialization=1
  state Idle
    x=0;
    t1=ts/timeStep;
  state State1
    x=1;
  state Wait
  (default) -> Idle
  Idle -> Idle [order 2]
  Wait -> Idle [order 2] : after(t1,'sec')
  Idle -> State1 [order 1] : [u>=1]
  State1 -> Idle [order 2] : [y==1]
  State1 -> Wait [order 1] : [u==0]
  Wait -> State1 [order 1] : [u==1]
  data: y input; u input; x output; ts input; timeStep constant double; t1 local

== stateflow chart smart_home/House Lighting Controler/Chart5 ==
  settings: updateMethod=DISCRETE  sampleTime=1  executeAtInitialization=1
  state Idle
    x=0;
    t1=ts/timeStep;
  state State1
    x=1;
  state Wait
  (default) -> Idle
  Idle -> Idle [order 2]
  Wait -> Idle [order 2] : after(t1,'sec')
  Idle -> State1 [order 1] : [u>=1]
  State1 -> Idle [order 2] : [y==1]
  State1 -> Wait [order 1] : [u==0]
  Wait -> State1 [order 1] : [u==1]
  data: y input; u input; x output; ts input; timeStep constant double; t1 local

== stateflow chart smart_home/Garden Lighting Controler/Chart6 ==
  settings: updateMethod=DISCRETE  sampleTime=1  executeAtInitialization=1
  state sun_up
    sunState=0;
  state sun_down
    sunState=1;
  (default) -> sun_up
  sun_up -> sun_down : [isSunrise]
  sun_down -> sun_up : [isSunset]
  data: isSunrise input; isSunset input; sunState output

== stateflow chart smart_home/House Lighting Controler/Chart6 ==
  settings: updateMethod=DISCRETE  sampleTime=1  executeAtInitialization=1
  state sun_up
    sunState=0;
  state sun_down
    sunState=1;
  (default) -> sun_up
  sun_up -> sun_down : [isSunrise]
  sun_down -> sun_up : [isSunset]
  data: isSunrise input; isSunset input; sunState output

== stateflow chart smart_home/Garage door/Chart ==
  settings: updateMethod=DISCRETE  sampleTime=1  executeAtInitialization=1
  state Idle
    x=0;
    t1=ts/timeStep;
  state State1
    x=1;
  state Wait
  (default) -> Idle
  Idle -> Idle [order 2]
  Wait -> Idle [order 2] : after(t1,'sec')
  Idle -> State1 [order 1] : [u>=1]
  State1 -> Idle [order 2] : [y==1]
  State1 -> Wait [order 1] : [u==0]
  Wait -> State1 [order 1] : [u==1]
  data: y input; u input; x output; ts input; timeStep constant double; t1 local

== stateflow chart smart_home/Watering Controler/Chart ==
  settings: updateMethod=DISCRETE  sampleTime=1  executeAtInitialization=1
  state Idle
    x=0;
    t1=ts/timeStep;
  state State1
    x=1;
  state Wait
  (default) -> Idle
  Idle -> Idle [order 2]
  Wait -> Idle [order 2] : after(t1,'sec')
  Idle -> State1 [order 1] : [u>=1]
  State1 -> Idle [order 2] : [y==1]
  State1 -> Wait [order 1] : [u==0]
  Wait -> State1 [order 1] : [u==1]
  data: y input; u input; x output; ts input; timeStep constant double; t1 local

== stateflow chart smart_home/Air Filter Controler ==
  state average
    filter_state=1;
  state good
    filter_state=0;
  (default) -> average
  average -> good : [average_quality]
  good -> average : [bad_quality]
  data: average_quality input; bad_quality input; filter_state output

== stateflow chart smart_home/Roof Windows Controler/Chart6 ==
  settings: updateMethod=DISCRETE  sampleTime=1  executeAtInitialization=1
  state sun_up
    sunState=false;
  state sun_down
    sunState=true;
  (default) -> sun_up
  sun_up -> sun_down : [isSunrise]
  sun_down -> sun_up : [isSunset]
  data: isSunrise input; isSunset input; sunState output
